simulink model "lab1"  (R2020b)
settings: Solver=VariableStepAuto  StartTime=0.0  StopTime=10.0  RelTol=1e-3
model workspace (MAT data in the model file):
  K1 = Simulink.Parameter
  K1.Value = 50
  K1.DataType = 'auto'
  K1.Dimensions = [1 1]
  K12 = Simulink.Parameter
  K12.Value = 20
  K12.DataType = 'auto'
  K12.Dimensions = [1 1]
  M1 = Simulink.Parameter
  M1.Value = 100
  M1.DataType = 'auto'
  M1.Dimensions = [1 1]
  M2 = Simulink.Parameter
  M2.Value = 20
  M2.DataType = 'auto'
  M2.Dimensions = [1 1]
  b = Simulink.Parameter
  b.Value = 50
  b.DataType = 'auto'
  b.Dimensions = [1 1]
settings Model: Creator=karth  LastModifiedBy=karth

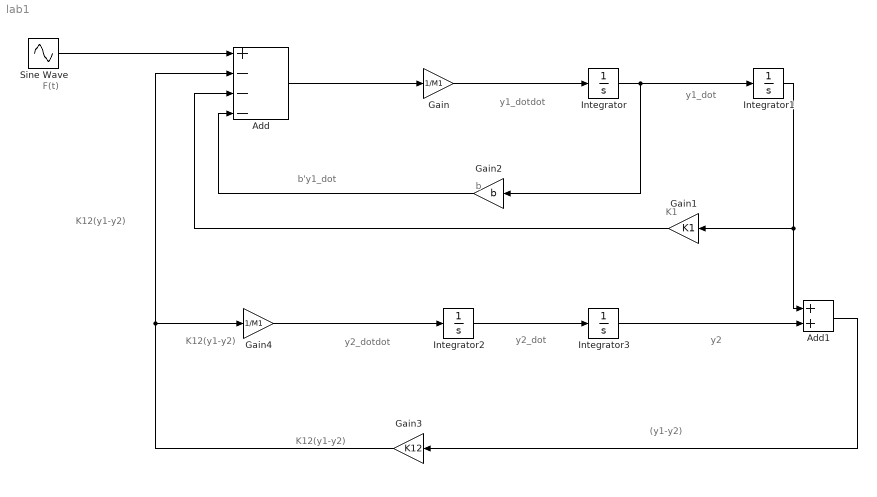
== system lab1 ==
  note: b'y1_dot
  note: b
  note: K1
  note: y2_dot
  note: y2
  note: K12(y1-y2)
  note: F(t)
  note: K12(y1-y2)
  note: K12(y1-y2)
  note: (y1-y2)
  note: y2_dotdot
  note: y1_dot
  note: y1_dotdot
  Add : Sum  Inputs=+---
  Add1 : Sum
  Gain : Gain  Gain=1/M1
  Gain1 : Gain  Gain=K1
  Gain2 : Gain  Gain=b
  Gain3 : Gain  Gain=K12
  Gain4 : Gain  Gain=1/M1
  Integrator{,1..3} (4 alike) : Integrator
  Sine Wave : Sin  Amplitude=2*pi*100  SampleTime=0
  wires:
  Sine Wave/1 -> Add/1
  Add/1 -> Gain/1
  Gain/1 -> Integrator/1
  Integrator/1 -> Gain2/1, Integrator1/1
  Gain4/1 -> Integrator2/1
  Integrator2/1 -> Integrator3/1
  Integrator3/1 -> Add1/2
  Add1/1 -> Gain3/1
  Gain2/1 -> Add/4
  Gain1/1 -> Add/3
  Gain3/1 -> Gain4/1, Add/2
  Integrator1/1 -> Gain1/1, Add1/1
